simulink model "iff_sim"  (R2019b)
settings: Solver=VariableStepAuto  StartTime=0.0  StopTime=T  FixedStep=0.001  MaxStep=0.01  RelTol=1e-3
values from neighbouring files (symbols this model uses):
  bsc = 17    [model.mat]
  d_r = [0.01 0.01 0.01 0.01 0.01 0.01]    [model.mat]
  Fi_b_z = in_rlb(12,1)    [fcn_s_rlb.m]    (also in fcn_s_rub.m = in_rub(12,1); model.mat = [0 2.09439510239 4.18879020479 1.0471975512 3.14159265359 5.)
  ka = 11860000    [model.mat]
  ksc = 179000    [model.mat]
  l_r = in_rlb(3,1)    [fcn_s_rlb.m]    (also in fcn_s_rub.m = in_rub(3,1); model.mat = [0.36 0.36 0.36 0.36 0.36 0.36])
  la00 = 0.061    [model.mat]
  linderiv = 0    [model.mat]
  O_lb = in_rlb(4:9,1)    [fcn_s_rlb.m]    (also in model.mat = [0 0 0 0 0 0])
  s_0 = s_d(:,:,1)    [iff_run.m]
  t_dist = 0.1    [model.mat]
  ts_noise = 0.00016    [model.mat]
  v_0 = v_d(:,:,1)    [iff_run.m]
  w_lb = in_rlb(11,1)    [fcn_s_rlb.m]    (also in model.mat = 0.195)
  W_lb = 0.205    [model.mat]
  w_ub = in_rub(11,1)    [fcn_s_rub.m]    (also in model.mat = 0.195)
  W_ub = 0.205    [model.mat]
undefined symbols (not defined in the file or in its folder): Kd, Kdiag, Ki, Kp, q_d, qt_d, qtt_d, t_d, X, Y, Z
libraries: nesl_utility x282, sm_lib x208, dspindex x30, simulink_extras x24, simulink x14, powerlib_meascontrol x1
(part 1 of 14)
settings Model: Creator=Vojta  LastModifiedBy=Tom
settings ExplorerConfigSet: InternalSimMechanicsExplorerSettings="<ExplorerConfiguration><canonicalview>default</canonicalview><AnimationSetting><BasePlaybackSpeed>1.0</BasePlaybackSpeed><PlaybackSpeedFactor>1.0</PlaybackSpeedFactor></AnimationSetting><TilePanel><TileInfo><Tiles Columns=\"1\" Count=\"1\" Rows=\"1\"><Column Weight=\"1\"/><Row Weight=\"1\"/><Tile Height=\"1\" Width=\"1\" X=\"0\" Y=\"0\"/></Tiles></TileInfo><SceneInfo><SceneViewer><BGColor><R>0.800000011920928955</R><G>0.800000011920928955</G><B>0.800000011920928955</B></BGColor><Camera><DoPerspective>off</DoPerspective><Position><X>0.685097738431936554</X><Y>0.708411390405585983</Y><Z>0.419719831436795587</Z></Position><Center><X>-5.89655776053188418e-05</X><Y>-0.000501993352412410943</Y><Z>0.252381535522246514</Z></Center><Up><X>-0.109250379592686409</X><Y>-0.127120209843101351</Y><Z>0.985852325050917688</Z></Up><ViewLimDist>1</ViewLimDist><YLim>0.288930054247379331</YLim><XLim>0.560223444501202317</XLim></Camera></SceneViewer></SceneInfo></TilePanel><MechEditorPanel><Cameras/><GfxPanelCameraMap/><VideoCreator><PlaybackSpeedRatio>1.0</PlaybackSpeedRatio><FrameRate>30</FrameRate><VideoFormat>Motion JPEG AVI</VideoFormat><FrameSize>auto</FrameSize></VideoCreator></MechEditorPanel></ExplorerConfiguration>"

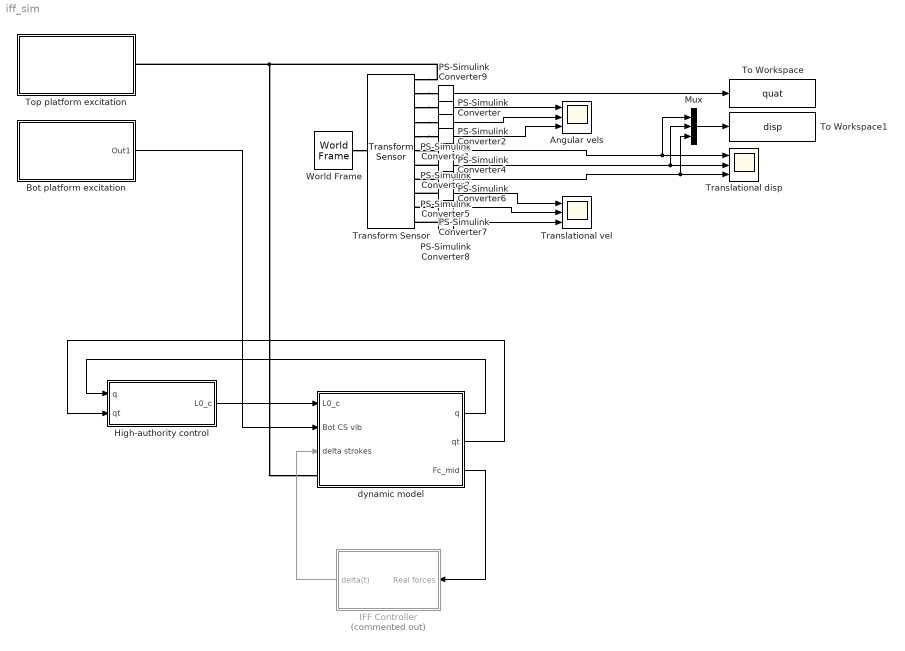
== system iff_sim ==
  Angular vels : Scope  NumInputPorts=3
  Bot platform excitation : Subsystem
  High-authority control : Subsystem
  IFF Controller : Subsystem  Commented=on
  Mux : Mux  Inputs=3
  PS-Simulink Converter{,1..9} (10 alike) : nesl_utility/PS-Simulink Converter  PhysicalDomain=network_engine_domain  SubClassName=ps_output  LeftPortType=input  RightPortType=output  PseudoPeriodic=off  Frequencies=[]  Unit=inherit  AffineConversion=off
  To Workspace : ToWorkspace  VariableName=quat  SaveFormat=Timeseries  SampleTime=-1
  To Workspace1 : ToWorkspace  VariableName=disp  SaveFormat=Timeseries  SampleTime=-1
  Top platform excitation : Subsystem
  Transform Sensor : sm_lib/Frames and Transforms/Transform Sensor  MeasurementFrame=World  SenseAngle=off  SenseAxis=off  SenseAngle1=off  SenseAngle2=off  SenseAngle3=off  SenseQ=on  SenseR=off  SenseOmegaX=on  SenseOmegaY=on  SenseOmegaZ=on  SenseOmega1=off  SenseOmega2=off  SenseOmega3=off  SenseQDot=off  SenseRDot=off  SenseAlphaX=off  SenseAlphaY=off  SenseAlphaZ=off  SenseAlpha1=off  SenseAlpha2=off  SenseAlpha3=off  SenseQDDot=off  SenseRDDot=off  SenseX=on  SenseY=on  SenseZ=on  SenseRad=off  SenseAzim=off  SenseDist=off  SenseInc=off  SenseXDot=on  SenseYDot=on  SenseZDot=on  SenseRadDot=off  SenseAzimDot=off  SenseDistDot=off  SenseIncDot=off  SenseXDDot=off  SenseYDDot=off  SenseZDDot=off  SenseRadDDot=off  SenseAzimDDot=off  SenseDistDDot=off  SenseIncDDot=off
  Translational vel : Scope  NumInputPorts=3
  Translational disp : Scope  NumInputPorts=3
  World Frame : sm_lib/Frames and Transforms/World Frame
  dynamic model : Subsystem
  wires:
  PS-Simulink Converter/1 -> Angular vels/1
  PS-Simulink Converter8/1 -> Translational vel/3
  PS-Simulink Converter7/1 -> Translational vel/2
  PS-Simulink Converter1/1 -> Angular vels/2
  PS-Simulink Converter6/1 -> Translational vel/1
  PS-Simulink Converter3/1 -> Mux/1, Translational disp/1
  PS-Simulink Converter5/1 -> Mux/3, Translational disp/3
  PS-Simulink Converter4/1 -> Mux/2, Translational disp/2
  PS-Simulink Converter2/1 -> Angular vels/3
  Bot platform excitation/1(Out1) -> dynamic model/2(Bot CS vib)
  dynamic model/1(q) -> High-authority control/1(q)
  dynamic model/2(qt) -> High-authority control/2(qt)
  High-authority control/1(L0_c) -> dynamic model/1(L0_c)
  dynamic model/3(Fc_mid) -> IFF Controller/1(Real forces)
  IFF Controller/1(delta(t)) -> dynamic model/3(delta strokes)
  PS-Simulink Converter9/1 -> To Workspace/1
  Mux/1 -> To Workspace1/1
  connections:
  Top platform excitation/RConn1 -- dynamic model/LConn1 -- Transform Sensor/RConn1
  World Frame/RConn1 -- Transform Sensor/LConn1
  Transform Sensor/RConn2 -- PS-Simulink Converter9/LConn1
  Transform Sensor/RConn3 -- PS-Simulink Converter/LConn1
  Transform Sensor/RConn4 -- PS-Simulink Converter1/LConn1
  Transform Sensor/RConn5 -- PS-Simulink Converter2/LConn1
  Transform Sensor/RConn6 -- PS-Simulink Converter3/LConn1
  PS-Simulink Converter4/LConn1 -- Transform Sensor/RConn7
  PS-Simulink Converter5/LConn1 -- Transform Sensor/RConn8
  PS-Simulink Converter6/LConn1 -- Transform Sensor/RConn9
  PS-Simulink Converter7/LConn1 -- Transform Sensor/RConn10
  PS-Simulink Converter8/LConn1 -- Transform Sensor/RConn11

== system iff_sim/Bot platform excitation ==
  Clock : Clock
  Constant : Constant  Value=0
  Constant1 : Constant  Value=0
  Manual Switch : ManualSwitch
  Manual Switch1 : ManualSwitch  CurrentSetting=0
  Scope : Scope
  Switch : Switch  Criteria=u2 > Threshold  Threshold=t_dist
  To Workspace : ToWorkspace  VariableName=bot_noise_out  SaveFormat=Timeseries  SampleTime=-1
  White noise : Subsystem
  Out1 : Outport
  wires:
  Clock/1 -> Manual Switch/1
  Manual Switch/1 -> Switch/2
  Switch/1 -> Scope/1, Manual Switch1/1
  Constant/1 -> Switch/3, Manual Switch/2
  Manual Switch1/1 -> To Workspace/1, Out1/1
  Constant1/1 -> Manual Switch1/2
  White noise/1(Out1) -> Switch/1

== system iff_sim/High-authority control ==
  q : Inport
  qt : Inport  Port=2
  CTC : Subsystem
  Constant : Constant
  Constant1 : Constant  Value=0
  Constant2 : Constant  Value=0
  Constant3 : Constant
  OL : Subsystem
  Sum : Sum  Inputs=|++
  Variant Source : VariantSource  ShowConditionOnBlock=on
  Variant Source1 : VariantSource  ShowConditionOnBlock=on
  L0_c : Outport
  wires:
  Variant Source1/1 -> CTC/Enable
  Constant2/1 -> Variant Source1/1
  Variant Source/1 -> OL/Enable
  CTC/1(L0_c) -> Sum/1
  Constant/1 -> Variant Source/1
  Constant3/1 -> Variant Source1/2
  OL/1(L0(t)) -> Sum/2
  q/1 -> CTC/1(q)
  Constant1/1 -> Variant Source/2
  qt/1 -> CTC/2(qt)
  Sum/1 -> L0_c/1

== system iff_sim/IFF Controller ==
  Real forces : Inport
  Basic IFF (real force) : Subsystem
  Derivative : Derivative
  Gain : Gain
  Gain2 : Gain  Gain=-1
  Highpass filt. (1 Hz cof) : powerlib_meascontrol/Filters/Second-Order Filter  FilterType=Highpass  Fo=1  Zeta=1  Ts=0  Initialize=off  Vac_Init="[0,  0,  60]"  Vdc_Init=0  PlotResponse=off  FreqRange=[0, 100, 10]
      settings: SourceProductName=Simscape Electrical  SourceProductBaseCode=PS
  Piezoactuator stroke [micron] : Scope
  Product : Product
  Real cable forces : Scope
  Scope1 : Scope
  g (max 65) : Constant  Value=ksc*Kdiag
  m to um : Gain  Gain=1e6
  delta(t) : Outport
  wires:
  Basic IFF (real force)/1(Stroke) -> m to um/1, delta(t)/1, Derivative/1
  Highpass filt. (1 Hz cof)/1 -> Basic IFF (real force)/1(Filtered force)
  m to um/1 -> Piezoactuator stroke [micron]/1
  Gain2/1 -> Scope1/1
  Derivative/1 -> Product/2
  Product/1 -> Gain2/1  "Energy dissipation by control [W]"
  Real forces/1 -> Product/1, Real cable forces/1, Highpass filt. (1 Hz cof)/1
  g (max 65)/1 -> Gain/1
  Gain/1 -> Basic IFF (real force)/2(IFF gain)

== system iff_sim/Top platform excitation ==
  Band-Limited White Noise : simulink/Sources/Band-Limited White Noise  Cov=top_noise  Ts=ts_noise  seed=[23559]
  Band-Limited White Noise1 : simulink/Sources/Band-Limited White Noise  Cov=top_noise  Ts=ts_noise  seed=[23558]
  Band-Limited White Noise2 : simulink/Sources/Band-Limited White Noise  Cov=top_noise  Ts=ts_noise  seed=[23557]
  Band-Limited White Noise3 : simulink/Sources/Band-Limited White Noise  Cov=top_noise  Ts=ts_noise  seed=[23541]
  Band-Limited White Noise4 : simulink/Sources/Band-Limited White Noise  Cov=top_noise  Ts=ts_noise  seed=[25342]
  Band-Limited White Noise5 : simulink/Sources/Band-Limited White Noise  Cov=top_noise  Ts=ts_noise  seed=[23543]
  Clock : Clock
  Constant : Constant  Value=0
  Demux : Demux  Outputs=6
  External Force and Torque : sm_lib/Forces and Torques/External Force and Torque  ForceResolutionFrame=World  EnableForceX=on  EnableForceY=on  EnableForceZ=on  EnableForce=off  TorqueResolutionFrame=World  EnableTorqueX=on  EnableTorqueY=on  EnableTorqueZ=on  EnableTorque=off
  Manual Switch : ManualSwitch
  Manual Switch1 : ManualSwitch  CurrentSetting=0
  Mux : Mux  Inputs=3
  Mux1 : Mux  Inputs=3
  Mux2 : Mux  Inputs=2
  Scope : Scope
  Simulink-PS Converter{,1..5} (6 alike) : nesl_utility/Simulink-PS Converter  PhysicalDomain=network_engine_domain  SubClassName=ps_input  LeftPortType=input  RightPortType=output  PseudoPeriodic=off  Frequencies=[]  NoiseDistribution=none  NoiseParameters=[]  Unit=1  AffineConversion=off  FilteringAndDerivatives=provide  SimscapeFilterOrder=1  InputFilterTimeConstant=0.001  UdotUserProvided=0
  Switch : Switch  Criteria=u2 > Threshold  Threshold=t_dist
  To Workspace : ToWorkspace  VariableName=top_noise_out  SaveFormat=Timeseries  SampleTime=-1
  Zero : Constant  Value=0  OutDataTypeStr=Inherit: Inherit via back propagation
  Top platform CS : PMIOPort  Side=Right
  wires:
  Constant/1 -> Manual Switch/2, Switch/3
  Mux/1 -> Mux2/2
  Manual Switch/1 -> Switch/2
  Clock/1 -> Manual Switch/1
  Band-Limited White Noise/1 -> Mux/1
  Band-Limited White Noise1/1 -> Mux/2
  Band-Limited White Noise2/1 -> Mux/3
  Zero/1 -> Manual Switch1/2
  Band-Limited White Noise5/1 -> Mux1/3
  Band-Limited White Noise4/1 -> Mux1/2
  Band-Limited White Noise3/1 -> Mux1/1
  Mux1/1 -> Mux2/1
  Mux2/1 -> To Workspace/1, Switch/1, Scope/1
  Switch/1 -> Manual Switch1/1
  Manual Switch1/1 -> Demux/1
  Demux/1 -> Simulink-PS Converter/1
  Demux/2 -> Simulink-PS Converter1/1
  Demux/3 -> Simulink-PS Converter2/1
  Demux/4 -> Simulink-PS Converter3/1
  Demux/5 -> Simulink-PS Converter4/1
  Demux/6 -> Simulink-PS Converter5/1
  connections:
  Top platform CS/RConn1 -- External Force and Torque/RConn1
  Simulink-PS Converter/RConn1 -- External Force and Torque/LConn1
  Simulink-PS Converter1/RConn1 -- External Force and Torque/LConn2
  Simulink-PS Converter2/RConn1 -- External Force and Torque/LConn3
  Simulink-PS Converter3/RConn1 -- External Force and Torque/LConn4
  Simulink-PS Converter4/RConn1 -- External Force and Torque/LConn5
  Simulink-PS Converter5/RConn1 -- External Force and Torque/LConn6

== system iff_sim/dynamic model ==
  L0_c : Inport
  Bot CS vib : Inport  Port=2
  delta strokes : Inport  Port=3
  Cable dynamics : Subsystem
  To Workspace : ToWorkspace  VariableName=l_c  SampleTime=-1
  To Workspace1 : ToWorkspace  VariableName=q  SampleTime=-1
  To Workspace2 : ToWorkspace  VariableName=qt  SampleTime=-1
  cables : Subsystem
  rods + bases : Subsystem  mask{s_r_0=s_0(:,1:6), v_r_0=v_0(:,1:6), s_ub_0=s_0(:,7), v_ub_0=v_0(:,7)}
  "s -> q" : MATLAB Function  TreatAsAtomicUnit=on
  scope l_c : Scope  Commented=on
  "v -> qt" : MATLAB Function  TreatAsAtomicUnit=on
  Top platform CS : PMIOPort  Side=Left
  q : Outport
  qt : Outport  Port=2
  Fc_mid : Outport  Port=3
  wires:
  rods + bases/1(s) -> "s -> q"/1(s)
  rods + bases/2(v) -> "v -> qt"/1(v)
  "s -> q"/1(q) -> To Workspace1/1, q/1
  "v -> qt"/1(qt) -> To Workspace2/1, qt/1
  cables/1(l_c) -> Cable dynamics/2(L0(t)), To Workspace/1, scope l_c/1
  Bot CS vib/1 -> rods + bases/1(Bot CS vib)
  L0_c/1 -> Cable dynamics/1(In1)
  delta strokes/1 -> Cable dynamics/3(In3)
  Cable dynamics/1(All cable forces) -> cables/1(F_c)
  Cable dynamics/2(Piezo cable forces) -> Fc_mid/1
  connections:
  rods + bases/RConn1 -- cables/LConn3 -- cables/LConn1
  cables/LConn13 -- cables/LConn15 -- cables/LConn36 -- cables/LConn10 -- rods + bases/RConn2
  rods + bases/RConn3 -- cables/LConn7 -- cables/LConn5
  cables/LConn17 -- cables/LConn19 -- cables/LConn28 -- cables/LConn2 -- rods + bases/RConn4
  rods + bases/RConn5 -- cables/LConn11 -- cables/LConn9
  cables/LConn21 -- cables/LConn23 -- cables/LConn32 -- cables/LConn6 -- rods + bases/RConn6
  cables/LConn16 -- cables/LConn18 -- cables/LConn34 -- cables/LConn4 -- rods + bases/RConn7
  rods + bases/RConn8 -- cables/LConn27 -- cables/LConn25
  cables/LConn20 -- cables/LConn22 -- cables/LConn26 -- cables/LConn8 -- rods + bases/RConn9
  rods + bases/RConn10 -- cables/LConn29 -- cables/LConn31
  cables/LConn14 -- cables/LConn24 -- cables/LConn30 -- cables/LConn12 -- rods + bases/RConn11
  rods + bases/RConn12 -- cables/LConn35 -- cables/LConn33
  Top platform CS/RConn1 -- rods + bases/LConn1

== system iff_sim/Bot platform excitation/White noise ==
  Band-Limited White Noise : simulink/Sources/Band-Limited White Noise  Cov=bot_noise  Ts=ts_noise  seed=[23341]
  Band-Limited White Noise1 : simulink/Sources/Band-Limited White Noise  Cov=bot_noise  Ts=ts_noise  seed=[23553]
  Band-Limited White Noise2 : simulink/Sources/Band-Limited White Noise  Cov=bot_noise  Ts=ts_noise  seed=[23552]
  Band-Limited White Noise3 : simulink/Sources/Band-Limited White Noise  Cov=bot_noise  Ts=ts_noise  seed=[23556]
  Band-Limited White Noise4 : simulink/Sources/Band-Limited White Noise  Cov=bot_noise  Ts=ts_noise  seed=[23555]
  Band-Limited White Noise5 : simulink/Sources/Band-Limited White Noise  Cov=bot_noise  Ts=ts_noise  seed=[23554]
  Mux : Mux  Inputs=3
  Mux1 : Mux  Inputs=3
  Mux2 : Mux  Inputs=2
  Out1 : Outport
  wires:
  Mux2/1 -> Out1/1
  Mux1/1 -> Mux2/1
  Band-Limited White Noise/1 -> Mux/1
  Band-Limited White Noise4/1 -> Mux1/2
  Band-Limited White Noise3/1 -> Mux1/1
  Band-Limited White Noise1/1 -> Mux/2
  Band-Limited White Noise2/1 -> Mux/3
  Band-Limited White Noise5/1 -> Mux1/3
  Mux/1 -> Mux2/2

== system iff_sim/High-authority control/CTC ==
  q : Inport
  qt : Inport  Port=2
  Enable : EnablePort
  Terminator : Terminator
  computed torque control : Subsystem
  inverse kinematics : Subsystem
  L0_c : Outport
  wires:
  inverse kinematics/2(qt_d) -> computed torque control/2(qt_d)
  inverse kinematics/1(q_d) -> computed torque control/1(q_d)
  computed torque control/2(L0_c) -> L0_c/1
  inverse kinematics/3(qtt_d) -> computed torque control/3(qtt_d)
  computed torque control/1(F_c) -> Terminator/1
  q/1 -> computed torque control/4(q)
  qt/1 -> computed torque control/5(qt)

== system iff_sim/High-authority control/OL ==
  Enable : EnablePort
  Desired cable free lengths : FromWorkspace  VariableName=L0_c
  Scope : Scope
  L0(t) : Outport
  wires:
  Desired cable free lengths/1 -> L0(t)/1, Scope/1

== system iff_sim/IFF Controller/Basic IFF (real force) ==
  Filtered force : Inport
  IFF gain : Inport  Port=2
  Gain : Gain  Gain=-1
  Integrator : Integrator
  Normalizing by specific stiffness : Gain  Gain=1/ksc
  Product : Product
  Stroke : Outport
  wires:
  Integrator/1 -> Product/1
  Normalizing by specific stiffness/1 -> Gain/1
  Filtered force/1 -> Integrator/1
  Gain/1 -> Stroke/1
  Product/1 -> Normalizing by specific stiffness/1
  IFF gain/1 -> Product/2

== system iff_sim/dynamic model/Cable dynamics ==
  In1 : Inport
  L0(t) : Inport  Port=2
  In3 : Inport  Port=3
  Constant : Constant  Value=ksc
  Hi-auth 1 : Selector  InputPortWidth=18  IndexOptions=Index vector (dialog)  Indices=[1 2 3 4 5 6]  OutputSizes=1
  Hi-auth 2 : Selector  InputPortWidth=18  IndexOptions=Index vector (dialog)  Indices=[13 14 15 16 17 18]  OutputSizes=1
  Mux : Mux  Inputs=3
  Real cable forces with spools and piezoactuators : Subsystem
  Real cable forces with spools only : Subsystem
  All cable forces : Outport
  Piezo cable forces : Outport  Port=2
  wires:
  Constant/1 -> Real cable forces with spools and piezoactuators/2(ksc), Real cable forces with spools only/2(ksc)
  Real cable forces with spools only/1(Fc(t)) -> Hi-auth 1/1, Hi-auth 2/1
  Hi-auth 1/1 -> Mux/1
  In1/1 -> Real cable forces with spools and piezoactuators/3(L0(t)), Real cable forces with spools only/1(L0(t))
  Real cable forces with spools and piezoactuators/1(Fc(t)) -> Piezo cable forces/1, Mux/2
  In3/1 -> Real cable forces with spools and piezoactuators/1(delta(t))
  Hi-auth 2/1 -> Mux/3
  L0(t)/1 -> Real cable forces with spools and piezoactuators/4(L(t)), Real cable forces with spools only/3(L(t))
  Mux/1 -> All cable forces/1

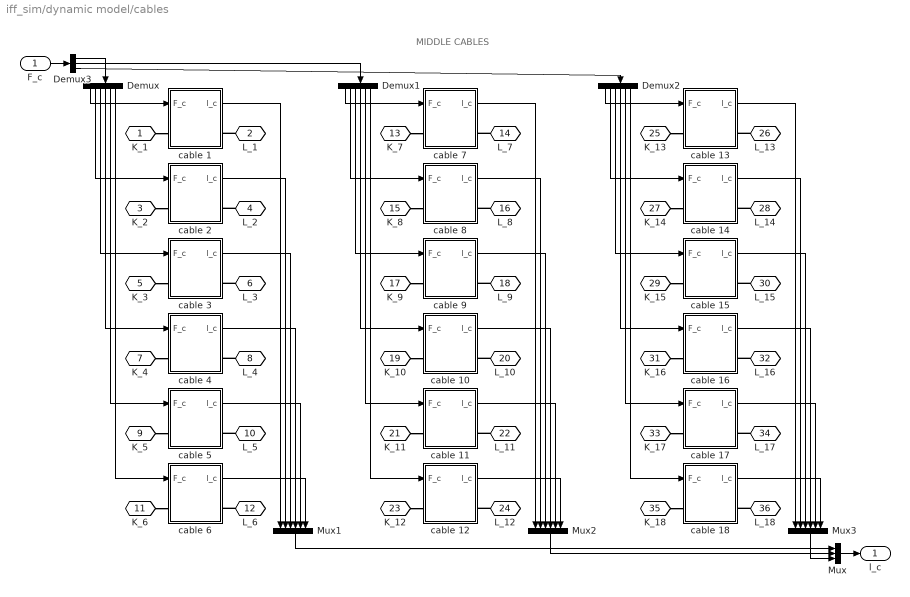
== system iff_sim/dynamic model/cables ==
  note: MIDDLE CABLES
  F_c : Inport
  Demux : Demux  Outputs=6
  Demux1 : Demux  Outputs=6
  Demux2 : Demux  Outputs=6
  Demux3 : Demux  Outputs=3
  Mux : Mux  Inputs=3
  Mux1 : Mux  Inputs=6
  Mux2 : Mux  Inputs=6
  Mux3 : Mux  Inputs=6
  cable 1 : Subsystem
  cable 10 : Subsystem
  cable 11 : Subsystem
  cable 12 : Subsystem
  cable 13 : Subsystem
  cable 14 : Subsystem
  cable 15 : Subsystem
  cable 16 : Subsystem
  cable 17 : Subsystem
  cable 18 : Subsystem
  cable 2 : Subsystem
  cable 3 : Subsystem
  cable 4 : Subsystem
  cable 5 : Subsystem
  cable 6 : Subsystem
  cable 7 : Subsystem
  cable 8 : Subsystem
  cable 9 : Subsystem
  K_1 : PMIOPort  Side=Left
  L_1 : PMIOPort  Port=2  Side=Left
  K_2 : PMIOPort  Port=3  Side=Left
  L_2 : PMIOPort  Port=4  Side=Left
  K_3 : PMIOPort  Port=5  Side=Left
  L_3 : PMIOPort  Port=6  Side=Left
  K_4 : PMIOPort  Port=7  Side=Left
  L_4 : PMIOPort  Port=8  Side=Left
  K_5 : PMIOPort  Port=9  Side=Left
  L_5 : PMIOPort  Port=10  Side=Left
  K_6 : PMIOPort  Port=11  Side=Left
  L_6 : PMIOPort  Port=12  Side=Left
  K_7 : PMIOPort  Port=13  Side=Left
  L_7 : PMIOPort  Port=14  Side=Left
  K_8 : PMIOPort  Port=15  Side=Left
  L_8 : PMIOPort  Port=16  Side=Left
  K_9 : PMIOPort  Port=17  Side=Left
  L_9 : PMIOPort  Port=18  Side=Left
  K_10 : PMIOPort  Port=19  Side=Left
  L_10 : PMIOPort  Port=20  Side=Left
  K_11 : PMIOPort  Port=21  Side=Left
  L_11 : PMIOPort  Port=22  Side=Left
  K_12 : PMIOPort  Port=23  Side=Left
  L_12 : PMIOPort  Port=24  Side=Left
  K_13 : PMIOPort  Port=25  Side=Left
  L_13 : PMIOPort  Port=26  Side=Left
  K_14 : PMIOPort  Port=27  Side=Left
  L_14 : PMIOPort  Port=28  Side=Left
  K_15 : PMIOPort  Port=29  Side=Left
  L_15 : PMIOPort  Port=30  Side=Left
  K_16 : PMIOPort  Port=31  Side=Left
  L_16 : PMIOPort  Port=32  Side=Left
  K_17 : PMIOPort  Port=33  Side=Left
  L_17 : PMIOPort  Port=34  Side=Left
  K_18 : PMIOPort  Port=35  Side=Left
  L_18 : PMIOPort  Port=36  Side=Left
  l_c : Outport
  wires:
  F_c/1 -> Demux3/1
  Mux/1 -> l_c/1
  Demux/1 -> cable 1/1(F_c)
  Demux/2 -> cable 2/1(F_c)
  Demux/3 -> cable 3/1(F_c)
  Demux/4 -> cable 4/1(F_c)
  Demux/5 -> cable 5/1(F_c)
  Demux/6 -> cable 6/1(F_c)
  cable 1/1(l_c) -> Mux1/1
  cable 2/1(l_c) -> Mux1/2
  cable 3/1(l_c) -> Mux1/3
  cable 4/1(l_c) -> Mux1/4
  cable 5/1(l_c) -> Mux1/5
  cable 6/1(l_c) -> Mux1/6
  cable 11/1(l_c) -> Mux2/5
  cable 8/1(l_c) -> Mux2/2
  Demux1/5 -> cable 11/1(F_c)
  Demux1/3 -> cable 9/1(F_c)
  Demux1/1 -> cable 7/1(F_c)
  Demux1/4 -> cable 10/1(F_c)
  cable 9/1(l_c) -> Mux2/3
  Demux1/2 -> cable 8/1(F_c)
  Demux1/6 -> cable 12/1(F_c)
  cable 7/1(l_c) -> Mux2/1
  cable 10/1(l_c) -> Mux2/4
  cable 12/1(l_c) -> Mux2/6
  cable 17/1(l_c) -> Mux3/5
  cable 14/1(l_c) -> Mux3/2
  Demux2/5 -> cable 17/1(F_c)
  Demux2/3 -> cable 15/1(F_c)
  Demux2/1 -> cable 13/1(F_c)
  Demux2/4 -> cable 16/1(F_c)
  cable 15/1(l_c) -> Mux3/3
  Demux2/2 -> cable 14/1(F_c)
  Demux2/6 -> cable 18/1(F_c)
  cable 13/1(l_c) -> Mux3/1
  cable 16/1(l_c) -> Mux3/4
  cable 18/1(l_c) -> Mux3/6
  Demux3/1 -> Demux/1
  Demux3/2 -> Demux1/1
  Demux3/3 -> Demux2/1
  Mux1/1 -> Mux/1
  Mux2/1 -> Mux/2
  Mux3/1 -> Mux/3
  connections:
  K_2/RConn1 -- cable 2/LConn1
  L_2/RConn1 -- cable 2/RConn1
  K_3/RConn1 -- cable 3/LConn1
  L_3/RConn1 -- cable 3/RConn1
  K_1/RConn1 -- cable 1/LConn1
  L_1/RConn1 -- cable 1/RConn1
  K_5/RConn1 -- cable 5/LConn1
  L_4/RConn1 -- cable 4/RConn1
  L_5/RConn1 -- cable 5/RConn1
  K_6/RConn1 -- cable 6/LConn1
  L_6/RConn1 -- cable 6/RConn1
  K_4/RConn1 -- cable 4/LConn1
  L_12/RConn1 -- cable 12/RConn1
  L_7/RConn1 -- cable 7/RConn1
  L_9/RConn1 -- cable 9/RConn1
  K_9/RConn1 -- cable 9/LConn1
  K_10/RConn1 -- cable 10/LConn1
  L_11/RConn1 -- cable 11/RConn1
  K_11/RConn1 -- cable 11/LConn1
  K_8/RConn1 -- cable 8/LConn1
  K_7/RConn1 -- cable 7/LConn1
  L_8/RConn1 -- cable 8/RConn1
  K_12/RConn1 -- cable 12/LConn1
  L_10/RConn1 -- cable 10/RConn1
  L_15/RConn1 -- cable 15/RConn1
  L_13/RConn1 -- cable 13/RConn1
  K_16/RConn1 -- cable 16/LConn1
  K_13/RConn1 -- cable 13/LConn1
  L_17/RConn1 -- cable 17/RConn1
  K_14/RConn1 -- cable 14/LConn1
  L_16/RConn1 -- cable 16/RConn1
  K_15/RConn1 -- cable 15/LConn1
  L_18/RConn1 -- cable 18/RConn1
  L_14/RConn1 -- cable 14/RConn1
  K_18/RConn1 -- cable 18/LConn1
  K_17/RConn1 -- cable 17/LConn1

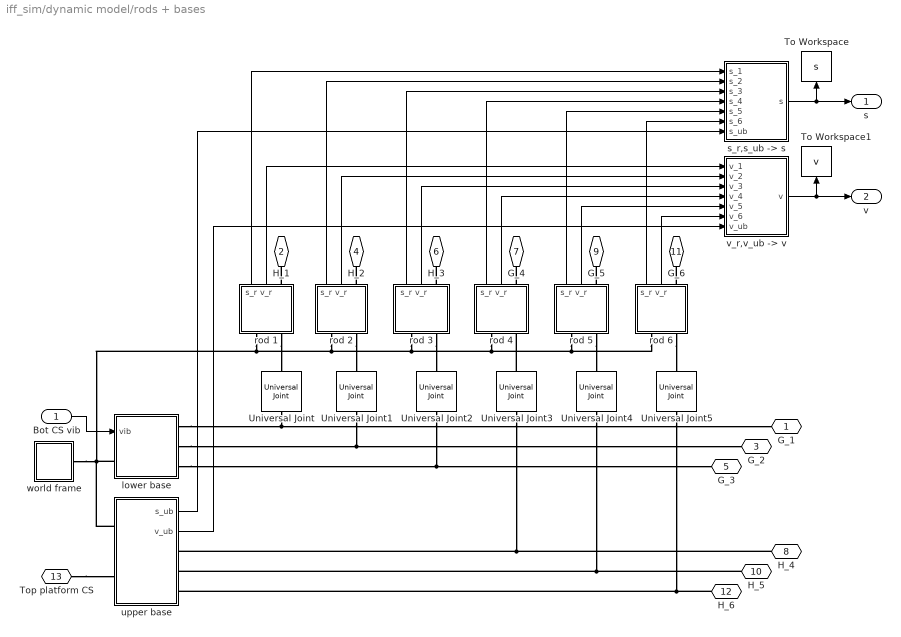
== system iff_sim/dynamic model/rods + bases ==
  Bot CS vib : Inport
  To Workspace : ToWorkspace  VariableName=s  SampleTime=-1
  To Workspace1 : ToWorkspace  VariableName=v  SampleTime=-1
  Universal Joint{,1..5} (6 alike) : sm_lib/Joints/Universal Joint  JointMode=Normal  SenseConstraintForce=off  SenseConstraintForceX=off  SenseConstraintForceY=off  SenseConstraintForceZ=off  SenseConstraintTorque=off  SenseConstraintTorqueX=off  SenseConstraintTorqueY=off  SenseConstraintTorqueZ=off  SenseTotalForce=off  SenseTotalForceX=off  SenseTotalForceY=off  SenseTotalForceZ=off  SenseTotalTorque=off  SenseTotalTorqueX=off  SenseTotalTorqueY=off  SenseTotalTorqueZ=off  CompositeWrenchDir=FollowerOnBase  CompositeWrenchFrame=BaseFrame  RxEquilibriumPosition=0  RxEquilibriumPositionUnits=deg  RxSpringStiffness=0  RxSpringStiffnessUnits=N*m/deg  RxDampingCoefficient=0  RxDampingCoefficientUnits=N*m/(deg/s)  RxTorqueActuationMode=NoTorque  RxMotionActuationMode=ComputedMotion  RxSensePosition=off  RxSenseVelocity=off  RxSenseAcceleration=off  RxSenseTorqueForce=off  RxSenseLowerLimitTorqueForce=off  RxSenseUpperLimitTorqueForce=off  RxLowerLimitSpecify=off  RxLowerLimitBound=-90  RxLowerLimitBoundUnits=deg  RxLowerLimitStiffness=1e4  RxLowerLimitStiffnessUnits=N*m/deg  RxLowerLimitDamping=10  RxLowerLimitDampingUnits=N*m/(deg/s)  RxLowerLimitTransitionRegionWidth=0.1  RxLowerLimitTransitionRegionWidthUnits=deg  RxUpperLimitSpecify=off  RxUpperLimitBound=90  RxUpperLimitBoundUnits=deg  RxUpperLimitStiffness=1e4  RxUpperLimitStiffnessUnits=N*m/deg  RxUpperLimitDamping=10  RxUpperLimitDampingUnits=N*m/(deg/s)  RxUpperLimitTransitionRegionWidth=0.1  RxUpperLimitTransitionRegionWidthUnits=deg  RxPositionTargetSpecify=off  RxPositionTargetPriority=High  RxPositionTargetValue=0  RxPositionTargetValueUnits=deg  RxVelocityTargetSpecify=off  RxVelocityTargetPriority=High  RxVelocityTargetValue=0  RxVelocityTargetValueUnits=deg/s  RyEquilibriumPosition=0  RyEquilibriumPositionUnits=deg  RySpringStiffness=0  RySpringStiffnessUnits=N*m/deg  RyDampingCoefficient=0  RyDampingCoefficientUnits=N*m/(deg/s)  RyTorqueActuationMode=NoTorque  RyMotionActuationMode=ComputedMotion  RySensePosition=off  RySenseVelocity=off  RySenseAcceleration=off  RySenseTorqueForce=off  RySenseLowerLimitTorqueForce=off  RySenseUpperLimitTorqueForce=off  RyLowerLimitSpecify=off  RyLowerLimitBound=-90  RyLowerLimitBoundUnits=deg  RyLowerLimitStiffness=1e4  RyLowerLimitStiffnessUnits=N*m/deg  RyLowerLimitDamping=10  RyLowerLimitDampingUnits=N*m/(deg/s)  RyLowerLimitTransitionRegionWidth=0.1  RyLowerLimitTransitionRegionWidthUnits=deg  RyUpperLimitSpecify=off  RyUpperLimitBound=90  RyUpperLimitBoundUnits=deg  RyUpperLimitStiffness=1e4  RyUpperLimitStiffnessUnits=N*m/deg  RyUpperLimitDamping=10  RyUpperLimitDampingUnits=N*m/(deg/s)  RyUpperLimitTransitionRegionWidth=0.1  RyUpperLimitTransitionRegionWidthUnits=deg  RyPositionTargetSpecify=off  RyPositionTargetPriority=High  RyPositionTargetValue=0  RyPositionTargetValueUnits=deg  RyVelocityTargetSpecify=off  RyVelocityTargetPriority=High  RyVelocityTargetValue=0  RyVelocityTargetValueUnits=deg/s
      settings: SourceProductName=Simscape Multibody
  lower base : Subsystem
  rod 1 : Subsystem  mask{r=1}
  rod 2 : Subsystem  mask{r=2}
  rod 3 : Subsystem  mask{r=3}
  rod 4 : Subsystem  mask{r=4}
  rod 5 : Subsystem  mask{r=5}
  rod 6 : Subsystem  mask{r=6}
  "s_r,s_ub -> s" : MATLAB Function  TreatAsAtomicUnit=on
  upper base : Subsystem
  "v_r,v_ub -> v" : MATLAB Function  TreatAsAtomicUnit=on
  world frame : Subsystem
  G_1 : PMIOPort  Side=Right
  H_1 : PMIOPort  Port=2  Side=Right
  G_2 : PMIOPort  Port=3  Side=Right
  H_2 : PMIOPort  Port=4  Side=Right
  G_3 : PMIOPort  Port=5  Side=Right
  H_3 : PMIOPort  Port=6  Side=Right
  G_4 : PMIOPort  Port=7  Side=Right
  H_4 : PMIOPort  Port=8  Side=Right
  G_5 : PMIOPort  Port=9  Side=Right
  H_5 : PMIOPort  Port=10  Side=Right
  G_6 : PMIOPort  Port=11  Side=Right
  H_6 : PMIOPort  Port=12  Side=Right
  Top platform CS : PMIOPort  Port=13  Side=Left
  s : Outport
  v : Outport  Port=2
  wires:
  rod 1/1(s_r) -> "s_r,s_ub -> s"/1(s_1)
  upper base/1(s_ub) -> "s_r,s_ub -> s"/7(s_ub)
  "v_r,v_ub -> v"/1(v) -> To Workspace1/1, v/1
  rod 1/2(v_r) -> "v_r,v_ub -> v"/1(v_1)
  upper base/2(v_ub) -> "v_r,v_ub -> v"/7(v_ub)
  rod 2/2(v_r) -> "v_r,v_ub -> v"/2(v_2)
  rod 2/1(s_r) -> "s_r,s_ub -> s"/2(s_2)
  rod 3/2(v_r) -> "v_r,v_ub -> v"/3(v_3)
  rod 3/1(s_r) -> "s_r,s_ub -> s"/3(s_3)
  rod 4/2(v_r) -> "v_r,v_ub -> v"/4(v_4)
  rod 4/1(s_r) -> "s_r,s_ub -> s"/4(s_4)
  rod 5/1(s_r) -> "s_r,s_ub -> s"/5(s_5)
  rod 5/2(v_r) -> "v_r,v_ub -> v"/5(v_5)
  rod 6/2(v_r) -> "v_r,v_ub -> v"/6(v_6)
  rod 6/1(s_r) -> "s_r,s_ub -> s"/6(s_6)
  "s_r,s_ub -> s"/1(s) -> To Workspace/1, s/1
  Bot CS vib/1 -> lower base/1(vib)
  connections:
  lower base/RConn1 -- Universal Joint/LConn1 -- G_1/RConn1
  lower base/RConn2 -- G_2/RConn1 -- Universal Joint1/LConn1
  lower base/RConn3 -- G_3/RConn1 -- Universal Joint2/LConn1
  Universal Joint3/LConn1 -- H_4/RConn1 -- upper base/RConn1
  Universal Joint4/LConn1 -- H_5/RConn1 -- upper base/RConn2
  H_6/RConn1 -- Universal Joint5/LConn1 -- upper base/RConn3
  rod 1/RConn1 -- H_1/RConn1
  rod 1/LConn2 -- Universal Joint/RConn1
  world frame/RConn1 -- rod 3/LConn1 -- rod 6/LConn1 -- rod 5/LConn1 -- rod 4/LConn1 -- rod 2/LConn1 -- rod 1/LConn1 -- lower base/LConn1 -- upper base/LConn1
  rod 2/RConn1 -- H_2/RConn1
  rod 2/LConn2 -- Universal Joint1/RConn1
  rod 3/LConn2 -- Universal Joint2/RConn1
  rod 3/RConn1 -- H_3/RConn1
  rod 4/RConn1 -- G_4/RConn1
  Universal Joint3/RConn1 -- rod 4/LConn2
  rod 5/RConn1 -- G_5/RConn1
  rod 5/LConn2 -- Universal Joint4/RConn1
  rod 6/RConn1 -- G_6/RConn1
  rod 6/LConn2 -- Universal Joint5/RConn1
  Top platform CS/RConn1 -- upper base/LConn2

== system iff_sim/High-authority control/CTC/computed torque control ==
  q_d : Inport
  qt_d : Inport  Port=2
  qtt_d : Inport  Port=3
  q : Inport  Port=4
  qt : Inport  Port=5
  Constant : Constant  Value=ksc
  Free cable lengths : Subsystem
  To Workspace : ToWorkspace  Commented=on  VariableName=s_ctc  SampleTime=-1
  To Workspace1 : ToWorkspace  Commented=on  VariableName=v_ctc  SampleTime=-1
  To Workspace2 : ToWorkspace  VariableName=F_c  SampleTime=-1
  To Workspace3 : ToWorkspace  VariableName=L0_c  SampleTime=-1
  bases + rods : Subsystem  mask{s_r_0=s_0(:,1:6), v_r_0=v_0(:,1:6), s_ub_0=s_0(:,7), v_ub_0=v_0(:,7)}
  desired cable vectors/ lengths : Subsystem
  "q_d,q -> a_ctc" : Subsystem
  scope F_c : Scope  Commented=on
  scope l_c,d : Scope  Commented=on
  scope q_ctc : Subsystem  Commented=on
  scope qt_ctc : Subsystem  Commented=on
  scope qtt_ctc : Subsystem  Commented=on
  F_c : Outport
  L0_c : Outport  Port=2
  wires:
  bases + rods/2(v_ctc) -> To Workspace1/1
  q_d/1 -> "q_d,q -> a_ctc"/1(q_d)
  "q_d,q -> a_ctc"/1(q_ctc) -> scope q_ctc/1(in), bases + rods/1(q_ctc)
  "q_d,q -> a_ctc"/3(qtt_ctc) -> scope qtt_ctc/1(in), bases + rods/3(qtt_ctc)
  bases + rods/1(s_ctc) -> To Workspace/1
  "q_d,q -> a_ctc"/2(qt_ctc) -> scope qt_ctc/1(in), bases + rods/2(qt_ctc)
  qt_d/1 -> "q_d,q -> a_ctc"/2(qt_d)
  qtt_d/1 -> "q_d,q -> a_ctc"/3(qtt_d)
  desired cable vectors/ lengths/1(l_c) -> Free cable lengths/1(Desired len), scope l_c,d/1
  q/1 -> "q_d,q -> a_ctc"/4(q)
  qt/1 -> "q_d,q -> a_ctc"/5(qt)
  desired cable vectors/ lengths/2(F_c) -> Free cable lengths/3(Desired F), scope F_c/1, F_c/1, To Workspace2/1
  Constant/1 -> Free cable lengths/2(Specific k)
  Free cable lengths/1(L0(t)) -> To Workspace3/1, L0_c/1
  connections:
  desired cable vectors/ lengths/LConn24 -- desired cable vectors/ lengths/LConn30 -- desired cable vectors/ lengths/LConn14 -- desired cable vectors/ lengths/LConn12 -- bases + rods/RConn11
  bases + rods/RConn3 -- desired cable vectors/ lengths/LConn5 -- desired cable vectors/ lengths/LConn7
  desired cable vectors/ lengths/LConn20 -- desired cable vectors/ lengths/LConn22 -- desired cable vectors/ lengths/LConn26 -- desired cable vectors/ lengths/LConn8 -- bases + rods/RConn9
  bases + rods/RConn5 -- desired cable vectors/ lengths/LConn9 -- desired cable vectors/ lengths/LConn11
  desired cable vectors/ lengths/LConn19 -- desired cable vectors/ lengths/LConn28 -- desired cable vectors/ lengths/LConn17 -- desired cable vectors/ lengths/LConn2 -- bases + rods/RConn4
  desired cable vectors/ lengths/LConn21 -- desired cable vectors/ lengths/LConn23 -- desired cable vectors/ lengths/LConn32 -- desired cable vectors/ lengths/LConn6 -- bases + rods/RConn6
  bases + rods/RConn10 -- desired cable vectors/ lengths/LConn29 -- desired cable vectors/ lengths/LConn31
  desired cable vectors/ lengths/LConn18 -- desired cable vectors/ lengths/LConn34 -- desired cable vectors/ lengths/LConn16 -- desired cable vectors/ lengths/LConn4 -- bases + rods/RConn7
  bases + rods/RConn8 -- desired cable vectors/ lengths/LConn25 -- desired cable vectors/ lengths/LConn27
  desired cable vectors/ lengths/LConn13 -- desired cable vectors/ lengths/LConn36 -- desired cable vectors/ lengths/LConn15 -- desired cable vectors/ lengths/LConn10 -- bases + rods/RConn2
  bases + rods/RConn12 -- desired cable vectors/ lengths/LConn33 -- desired cable vectors/ lengths/LConn35
  bases + rods/RConn1 -- desired cable vectors/ lengths/LConn1 -- desired cable vectors/ lengths/LConn3

== system iff_sim/High-authority control/CTC/inverse kinematics ==
  Clock : Clock
  To Workspace : ToWorkspace  VariableName=t  SampleTime=-1
  "t -> q_d" : Subsystem  mask{Q_d=q_d}
  "t -> qt_d" : Subsystem  mask{Q_d=qt_d}
  "t -> qtt_d" : Subsystem  mask{Q_d=qtt_d}
  q_d : Outport
  qt_d : Outport  Port=2
  qtt_d : Outport  Port=3
  wires:
  "t -> q_d"/1(Q_d) -> q_d/1
  Clock/1 -> "t -> qt_d"/1(t), To Workspace/1, "t -> qtt_d"/1(t), "t -> q_d"/1(t)
  "t -> qt_d"/1(Q_d) -> qt_d/1
  "t -> qtt_d"/1(Q_d) -> qtt_d/1

== system iff_sim/dynamic model/Cable dynamics/Real cable forces with spools and piezoactuators ==
  delta(t) : Inport  PortDimensions=6
  ksc : Inport  Port=2
  L0(t) : Inport  Port=3
  L(t) : Inport  Port=4
  "Actuator free length, zero voltage" : Constant  Value=la00
  Actuator stiffness : Constant  Value=ka
  Cable specific damping : Constant  Value=bsc
  Derivative1 : Subsystem
  Divide : Product  Inputs=*/*
  Divide1 : Product  Inputs=*/
  Divide2 : Product  Inputs=**/
  Lo-auth : Selector  InputPortWidth=18  IndexOptions=Index vector (dialog)  Indices=[7 8 9 10 11 12]  OutputSizes=1
  Lo-auth1 : Selector  InputPortWidth=18  IndexOptions=Index vector (dialog)  Indices=[7 8 9 10 11 12]  OutputSizes=1
  Product : Product
  Scope : Scope
  Scope1 : Scope
  Sum : Sum  Inputs=++-
  Sum1 : Sum  Inputs=+|+
  Sum2 : Sum  Inputs=|-+
  Sum3 : Sum  Inputs=+|+
  Sum5 : Sum  Inputs=+|-
  Sum6 : Sum  Inputs=|+-
  Fc(t) : Outport  PortDimensions=6
  wires:
  Lo-auth1/1 -> Sum2/2, Sum/3, Sum5/1
  Lo-auth/1 -> Sum6/1, Sum/1
  Sum6/1 -> Derivative1/1(In1)
  Divide/1 -> Scope/1, Sum1/1  "Damping force"
  Derivative1/1(Out1) -> Divide/3
  Sum5/1 -> Divide/2
  Cable specific damping/1 -> Divide/1
  Sum1/1 -> Fc(t)/1
  Sum/1 -> Product/1
  delta(t)/1 -> Sum6/2, Sum/2
  Sum3/1 -> Divide2/3
  L(t)/1 -> Lo-auth/1
  Product/1 -> Sum1/2, Scope1/1  "Stiffness force"
  "Actuator free length, zero voltage"/1 -> Sum2/1, Sum5/2
  Divide2/1 -> Product/2  "Total stiffness of the element"
  ksc/1 -> Divide1/1
  Sum2/1 -> Divide1/2  "lc0(t)"
  L0(t)/1 -> Lo-auth1/1
  Actuator stiffness/1 -> Sum3/1, Divide2/1
  Divide1/1 -> Sum3/2, Divide2/2  "kc(t)"

== system iff_sim/dynamic model/Cable dynamics/Real cable forces with spools only ==
  L0(t) : Inport
  ksc : Inport  Port=2
  L(t) : Inport  Port=3
  Cable specific damping : Constant  Value=bsc
  Derivative : Subsystem
  Divide : Product  Inputs=*/*
  Divide1 : Product  Inputs=/**
  Scope : Scope
  Scope1 : Scope
  Sum1 : Sum  Inputs=+|+
  Sum3 : Sum  Inputs=|-+
  Fc(t) : Outport
  wires:
  ksc/1 -> Divide1/3
  Sum3/1 -> Divide1/2
  L0(t)/1 -> Sum3/1, Divide/2, Divide1/1
  L(t)/1 -> Derivative/1(In1), Sum3/2
  Cable specific damping/1 -> Divide/1
  Divide/1 -> Sum1/1, Scope/1  "Damping force"
  Divide1/1 -> Scope1/1, Sum1/2  "Stiffness force"
  Sum1/1 -> Fc(t)/1
  Derivative/1(Out1) -> Divide/3

== system iff_sim/dynamic model/cables/cable 1 ==
  F_c : Inport
  Internal Force : sm_lib/Forces and Torques/Internal Force
      settings: SourceProductName=Simscape Multibody  SourceProductBaseCode=MS
  PS-Simulink Converter3 : nesl_utility/PS-Simulink Converter  PhysicalDomain=network_engine_domain  SubClassName=ps_output  LeftPortType=input  RightPortType=output  PseudoPeriodic=off  Frequencies=[]  Unit=m  AffineConversion=off
  Simulink-PS Converter : nesl_utility/Simulink-PS Converter  PhysicalDomain=network_engine_domain  SubClassName=ps_input  LeftPortType=input  RightPortType=output  PseudoPeriodic=off  Frequencies=[]  NoiseDistribution=none  NoiseParameters=[]  Unit=N  AffineConversion=off  FilteringAndDerivatives=provide  SimscapeFilterOrder=1  InputFilterTimeConstant=0.001  UdotUserProvided=0
  Transform Sensor : sm_lib/Frames and Transforms/Transform Sensor  MeasurementFrame=World  SenseAngle=off  SenseAxis=off  SenseAngle1=off  SenseAngle2=off  SenseAngle3=off  SenseQ=off  SenseR=off  SenseOmegaX=off  SenseOmegaY=off  SenseOmegaZ=off  SenseOmega1=off  SenseOmega2=off  SenseOmega3=off  SenseQDot=off  SenseRDot=off  SenseAlphaX=off  SenseAlphaY=off  SenseAlphaZ=off  SenseAlpha1=off  SenseAlpha2=off  SenseAlpha3=off  SenseQDDot=off  SenseRDDot=off  SenseX=off  SenseY=off  SenseZ=off  SenseRad=off  SenseAzim=off  SenseDist=on  SenseInc=off  SenseXDot=off  SenseYDot=off  SenseZDot=off  SenseRadDot=off  SenseAzimDot=off  SenseDistDot=off  SenseIncDot=off  SenseXDDot=off  SenseYDDot=off  SenseZDDot=off  SenseRadDDot=off  SenseAzimDDot=off  SenseDistDDot=off  SenseIncDDot=off
  force orientation : Gain  Gain=-1
  K_c : PMIOPort  Side=Left
  L_c : PMIOPort  Port=2  Side=Right
  l_c : Outport
  wires:
  PS-Simulink Converter3/1 -> l_c/1
  F_c/1 -> force orientation/1
  force orientation/1 -> Simulink-PS Converter/1
  connections:
  PS-Simulink Converter3/LConn1 -- Transform Sensor/RConn2
  L_c/RConn1 -- Transform Sensor/RConn1 -- Internal Force/RConn1
  Internal Force/LConn1 -- K_c/RConn1 -- Transform Sensor/LConn1
  Simulink-PS Converter/RConn1 -- Internal Force/LConn2

== system iff_sim/dynamic model/cables/cable 10 ==
  F_c : Inport
  Internal Force : sm_lib/Forces and Torques/Internal Force
      settings: SourceProductName=Simscape Multibody  SourceProductBaseCode=MS
  PS-Simulink Converter3 : nesl_utility/PS-Simulink Converter  PhysicalDomain=network_engine_domain  SubClassName=ps_output  LeftPortType=input  RightPortType=output  PseudoPeriodic=off  Frequencies=[]  Unit=m  AffineConversion=off
  Simulink-PS Converter : nesl_utility/Simulink-PS Converter  PhysicalDomain=network_engine_domain  SubClassName=ps_input  LeftPortType=input  RightPortType=output  PseudoPeriodic=off  Frequencies=[]  NoiseDistribution=none  NoiseParameters=[]  Unit=N  AffineConversion=off  FilteringAndDerivatives=provide  SimscapeFilterOrder=1  InputFilterTimeConstant=0.001  UdotUserProvided=0
  Transform Sensor : sm_lib/Frames and Transforms/Transform Sensor  MeasurementFrame=World  SenseAngle=off  SenseAxis=off  SenseAngle1=off  SenseAngle2=off  SenseAngle3=off  SenseQ=off  SenseR=off  SenseOmegaX=off  SenseOmegaY=off  SenseOmegaZ=off  SenseOmega1=off  SenseOmega2=off  SenseOmega3=off  SenseQDot=off  SenseRDot=off  SenseAlphaX=off  SenseAlphaY=off  SenseAlphaZ=off  SenseAlpha1=off  SenseAlpha2=off  SenseAlpha3=off  SenseQDDot=off  SenseRDDot=off  SenseX=off  SenseY=off  SenseZ=off  SenseRad=off  SenseAzim=off  SenseDist=on  SenseInc=off  SenseXDot=off  SenseYDot=off  SenseZDot=off  SenseRadDot=off  SenseAzimDot=off  SenseDistDot=off  SenseIncDot=off  SenseXDDot=off  SenseYDDot=off  SenseZDDot=off  SenseRadDDot=off  SenseAzimDDot=off  SenseDistDDot=off  SenseIncDDot=off
  force orientation : Gain  Gain=-1
  K_c : PMIOPort  Side=Left
  L_c : PMIOPort  Port=2  Side=Right
  l_c : Outport
  wires:
  PS-Simulink Converter3/1 -> l_c/1
  F_c/1 -> force orientation/1
  force orientation/1 -> Simulink-PS Converter/1
  connections:
  PS-Simulink Converter3/LConn1 -- Transform Sensor/RConn2
  L_c/RConn1 -- Transform Sensor/RConn1 -- Internal Force/RConn1
  Internal Force/LConn1 -- K_c/RConn1 -- Transform Sensor/LConn1
  Simulink-PS Converter/RConn1 -- Internal Force/LConn2

== system iff_sim/dynamic model/cables/cable 11 ==
  F_c : Inport
  Internal Force : sm_lib/Forces and Torques/Internal Force
      settings: SourceProductName=Simscape Multibody  SourceProductBaseCode=MS
  PS-Simulink Converter3 : nesl_utility/PS-Simulink Converter  PhysicalDomain=network_engine_domain  SubClassName=ps_output  LeftPortType=input  RightPortType=output  PseudoPeriodic=off  Frequencies=[]  Unit=m  AffineConversion=off
  Simulink-PS Converter : nesl_utility/Simulink-PS Converter  PhysicalDomain=network_engine_domain  SubClassName=ps_input  LeftPortType=input  RightPortType=output  PseudoPeriodic=off  Frequencies=[]  NoiseDistribution=none  NoiseParameters=[]  Unit=N  AffineConversion=off  FilteringAndDerivatives=provide  SimscapeFilterOrder=1  InputFilterTimeConstant=0.001  UdotUserProvided=0
  Transform Sensor : sm_lib/Frames and Transforms/Transform Sensor  MeasurementFrame=World  SenseAngle=off  SenseAxis=off  SenseAngle1=off  SenseAngle2=off  SenseAngle3=off  SenseQ=off  SenseR=off  SenseOmegaX=off  SenseOmegaY=off  SenseOmegaZ=off  SenseOmega1=off  SenseOmega2=off  SenseOmega3=off  SenseQDot=off  SenseRDot=off  SenseAlphaX=off  SenseAlphaY=off  SenseAlphaZ=off  SenseAlpha1=off  SenseAlpha2=off  SenseAlpha3=off  SenseQDDot=off  SenseRDDot=off  SenseX=off  SenseY=off  SenseZ=off  SenseRad=off  SenseAzim=off  SenseDist=on  SenseInc=off  SenseXDot=off  SenseYDot=off  SenseZDot=off  SenseRadDot=off  SenseAzimDot=off  SenseDistDot=off  SenseIncDot=off  SenseXDDot=off  SenseYDDot=off  SenseZDDot=off  SenseRadDDot=off  SenseAzimDDot=off  SenseDistDDot=off  SenseIncDDot=off
  force orientation : Gain  Gain=-1
  K_c : PMIOPort  Side=Left
  L_c : PMIOPort  Port=2  Side=Right
  l_c : Outport
  wires:
  PS-Simulink Converter3/1 -> l_c/1
  F_c/1 -> force orientation/1
  force orientation/1 -> Simulink-PS Converter/1
  connections:
  PS-Simulink Converter3/LConn1 -- Transform Sensor/RConn2
  L_c/RConn1 -- Transform Sensor/RConn1 -- Internal Force/RConn1
  Internal Force/LConn1 -- K_c/RConn1 -- Transform Sensor/LConn1
  Simulink-PS Converter/RConn1 -- Internal Force/LConn2

== system iff_sim/dynamic model/cables/cable 12 ==
  F_c : Inport
  Internal Force : sm_lib/Forces and Torques/Internal Force
      settings: SourceProductName=Simscape Multibody  SourceProductBaseCode=MS
  PS-Simulink Converter3 : nesl_utility/PS-Simulink Converter  PhysicalDomain=network_engine_domain  SubClassName=ps_output  LeftPortType=input  RightPortType=output  PseudoPeriodic=off  Frequencies=[]  Unit=m  AffineConversion=off
  Simulink-PS Converter : nesl_utility/Simulink-PS Converter  PhysicalDomain=network_engine_domain  SubClassName=ps_input  LeftPortType=input  RightPortType=output  PseudoPeriodic=off  Frequencies=[]  NoiseDistribution=none  NoiseParameters=[]  Unit=N  AffineConversion=off  FilteringAndDerivatives=provide  SimscapeFilterOrder=1  InputFilterTimeConstant=0.001  UdotUserProvided=0
  Transform Sensor : sm_lib/Frames and Transforms/Transform Sensor  MeasurementFrame=World  SenseAngle=off  SenseAxis=off  SenseAngle1=off  SenseAngle2=off  SenseAngle3=off  SenseQ=off  SenseR=off  SenseOmegaX=off  SenseOmegaY=off  SenseOmegaZ=off  SenseOmega1=off  SenseOmega2=off  SenseOmega3=off  SenseQDot=off  SenseRDot=off  SenseAlphaX=off  SenseAlphaY=off  SenseAlphaZ=off  SenseAlpha1=off  SenseAlpha2=off  SenseAlpha3=off  SenseQDDot=off  SenseRDDot=off  SenseX=off  SenseY=off  SenseZ=off  SenseRad=off  SenseAzim=off  SenseDist=on  SenseInc=off  SenseXDot=off  SenseYDot=off  SenseZDot=off  SenseRadDot=off  SenseAzimDot=off  SenseDistDot=off  SenseIncDot=off  SenseXDDot=off  SenseYDDot=off  SenseZDDot=off  SenseRadDDot=off  SenseAzimDDot=off  SenseDistDDot=off  SenseIncDDot=off
  force orientation : Gain  Gain=-1
  K_c : PMIOPort  Side=Left
  L_c : PMIOPort  Port=2  Side=Right
  l_c : Outport
  wires:
  PS-Simulink Converter3/1 -> l_c/1
  F_c/1 -> force orientation/1
  force orientation/1 -> Simulink-PS Converter/1
  connections:
  PS-Simulink Converter3/LConn1 -- Transform Sensor/RConn2
  L_c/RConn1 -- Transform Sensor/RConn1 -- Internal Force/RConn1
  Internal Force/LConn1 -- K_c/RConn1 -- Transform Sensor/LConn1
  Simulink-PS Converter/RConn1 -- Internal Force/LConn2

== system iff_sim/dynamic model/cables/cable 13 ==
  F_c : Inport
  Internal Force : sm_lib/Forces and Torques/Internal Force
      settings: SourceProductName=Simscape Multibody  SourceProductBaseCode=MS
  PS-Simulink Converter3 : nesl_utility/PS-Simulink Converter  PhysicalDomain=network_engine_domain  SubClassName=ps_output  LeftPortType=input  RightPortType=output  PseudoPeriodic=off  Frequencies=[]  Unit=m  AffineConversion=off
  Simulink-PS Converter : nesl_utility/Simulink-PS Converter  PhysicalDomain=network_engine_domain  SubClassName=ps_input  LeftPortType=input  RightPortType=output  PseudoPeriodic=off  Frequencies=[]  NoiseDistribution=none  NoiseParameters=[]  Unit=N  AffineConversion=off  FilteringAndDerivatives=provide  SimscapeFilterOrder=1  InputFilterTimeConstant=0.001  UdotUserProvided=0
  Transform Sensor : sm_lib/Frames and Transforms/Transform Sensor  MeasurementFrame=World  SenseAngle=off  SenseAxis=off  SenseAngle1=off  SenseAngle2=off  SenseAngle3=off  SenseQ=off  SenseR=off  SenseOmegaX=off  SenseOmegaY=off  SenseOmegaZ=off  SenseOmega1=off  SenseOmega2=off  SenseOmega3=off  SenseQDot=off  SenseRDot=off  SenseAlphaX=off  SenseAlphaY=off  SenseAlphaZ=off  SenseAlpha1=off  SenseAlpha2=off  SenseAlpha3=off  SenseQDDot=off  SenseRDDot=off  SenseX=off  SenseY=off  SenseZ=off  SenseRad=off  SenseAzim=off  SenseDist=on  SenseInc=off  SenseXDot=off  SenseYDot=off  SenseZDot=off  SenseRadDot=off  SenseAzimDot=off  SenseDistDot=off  SenseIncDot=off  SenseXDDot=off  SenseYDDot=off  SenseZDDot=off  SenseRadDDot=off  SenseAzimDDot=off  SenseDistDDot=off  SenseIncDDot=off
  force orientation : Gain  Gain=-1
  K_c : PMIOPort  Side=Left
  L_c : PMIOPort  Port=2  Side=Right
  l_c : Outport
  wires:
  PS-Simulink Converter3/1 -> l_c/1
  F_c/1 -> force orientation/1
  force orientation/1 -> Simulink-PS Converter/1
  connections:
  PS-Simulink Converter3/LConn1 -- Transform Sensor/RConn2
  L_c/RConn1 -- Transform Sensor/RConn1 -- Internal Force/RConn1
  Internal Force/LConn1 -- K_c/RConn1 -- Transform Sensor/LConn1
  Simulink-PS Converter/RConn1 -- Internal Force/LConn2

== system iff_sim/dynamic model/cables/cable 14 ==
  F_c : Inport
  Internal Force : sm_lib/Forces and Torques/Internal Force
      settings: SourceProductName=Simscape Multibody  SourceProductBaseCode=MS
  PS-Simulink Converter3 : nesl_utility/PS-Simulink Converter  PhysicalDomain=network_engine_domain  SubClassName=ps_output  LeftPortType=input  RightPortType=output  PseudoPeriodic=off  Frequencies=[]  Unit=m  AffineConversion=off
  Simulink-PS Converter : nesl_utility/Simulink-PS Converter  PhysicalDomain=network_engine_domain  SubClassName=ps_input  LeftPortType=input  RightPortType=output  PseudoPeriodic=off  Frequencies=[]  NoiseDistribution=none  NoiseParameters=[]  Unit=N  AffineConversion=off  FilteringAndDerivatives=provide  SimscapeFilterOrder=1  InputFilterTimeConstant=0.001  UdotUserProvided=0
  Transform Sensor : sm_lib/Frames and Transforms/Transform Sensor  MeasurementFrame=World  SenseAngle=off  SenseAxis=off  SenseAngle1=off  SenseAngle2=off  SenseAngle3=off  SenseQ=off  SenseR=off  SenseOmegaX=off  SenseOmegaY=off  SenseOmegaZ=off  SenseOmega1=off  SenseOmega2=off  SenseOmega3=off  SenseQDot=off  SenseRDot=off  SenseAlphaX=off  SenseAlphaY=off  SenseAlphaZ=off  SenseAlpha1=off  SenseAlpha2=off  SenseAlpha3=off  SenseQDDot=off  SenseRDDot=off  SenseX=off  SenseY=off  SenseZ=off  SenseRad=off  SenseAzim=off  SenseDist=on  SenseInc=off  SenseXDot=off  SenseYDot=off  SenseZDot=off  SenseRadDot=off  SenseAzimDot=off  SenseDistDot=off  SenseIncDot=off  SenseXDDot=off  SenseYDDot=off  SenseZDDot=off  SenseRadDDot=off  SenseAzimDDot=off  SenseDistDDot=off  SenseIncDDot=off
  force orientation : Gain  Gain=-1
  K_c : PMIOPort  Side=Left
  L_c : PMIOPort  Port=2  Side=Right
  l_c : Outport
  wires:
  PS-Simulink Converter3/1 -> l_c/1
  F_c/1 -> force orientation/1
  force orientation/1 -> Simulink-PS Converter/1
  connections:
  PS-Simulink Converter3/LConn1 -- Transform Sensor/RConn2
  L_c/RConn1 -- Transform Sensor/RConn1 -- Internal Force/RConn1
  Internal Force/LConn1 -- K_c/RConn1 -- Transform Sensor/LConn1
  Simulink-PS Converter/RConn1 -- Internal Force/LConn2

== system iff_sim/dynamic model/cables/cable 15 ==
  F_c : Inport
  Internal Force : sm_lib/Forces and Torques/Internal Force
      settings: SourceProductName=Simscape Multibody  SourceProductBaseCode=MS
  PS-Simulink Converter3 : nesl_utility/PS-Simulink Converter  PhysicalDomain=network_engine_domain  SubClassName=ps_output  LeftPortType=input  RightPortType=output  PseudoPeriodic=off  Frequencies=[]  Unit=m  AffineConversion=off
  Simulink-PS Converter : nesl_utility/Simulink-PS Converter  PhysicalDomain=network_engine_domain  SubClassName=ps_input  LeftPortType=input  RightPortType=output  PseudoPeriodic=off  Frequencies=[]  NoiseDistribution=none  NoiseParameters=[]  Unit=N  AffineConversion=off  FilteringAndDerivatives=provide  SimscapeFilterOrder=1  InputFilterTimeConstant=0.001  UdotUserProvided=0
  Transform Sensor : sm_lib/Frames and Transforms/Transform Sensor  MeasurementFrame=World  SenseAngle=off  SenseAxis=off  SenseAngle1=off  SenseAngle2=off  SenseAngle3=off  SenseQ=off  SenseR=off  SenseOmegaX=off  SenseOmegaY=off  SenseOmegaZ=off  SenseOmega1=off  SenseOmega2=off  SenseOmega3=off  SenseQDot=off  SenseRDot=off  SenseAlphaX=off  SenseAlphaY=off  SenseAlphaZ=off  SenseAlpha1=off  SenseAlpha2=off  SenseAlpha3=off  SenseQDDot=off  SenseRDDot=off  SenseX=off  SenseY=off  SenseZ=off  SenseRad=off  SenseAzim=off  SenseDist=on  SenseInc=off  SenseXDot=off  SenseYDot=off  SenseZDot=off  SenseRadDot=off  SenseAzimDot=off  SenseDistDot=off  SenseIncDot=off  SenseXDDot=off  SenseYDDot=off  SenseZDDot=off  SenseRadDDot=off  SenseAzimDDot=off  SenseDistDDot=off  SenseIncDDot=off
  force orientation : Gain  Gain=-1
  K_c : PMIOPort  Side=Left
  L_c : PMIOPort  Port=2  Side=Right
  l_c : Outport
  wires:
  PS-Simulink Converter3/1 -> l_c/1
  F_c/1 -> force orientation/1
  force orientation/1 -> Simulink-PS Converter/1
  connections:
  PS-Simulink Converter3/LConn1 -- Transform Sensor/RConn2
  L_c/RConn1 -- Transform Sensor/RConn1 -- Internal Force/RConn1
  Internal Force/LConn1 -- K_c/RConn1 -- Transform Sensor/LConn1
  Simulink-PS Converter/RConn1 -- Internal Force/LConn2
